simulink model "Energisense"  (R2025a)
settings: Solver=VariableStepAuto  StartTime=0.0  StopTime=100  RelTol=1e-3
settings Model: Creator=Aryan  LastModifiedBy=Aryan

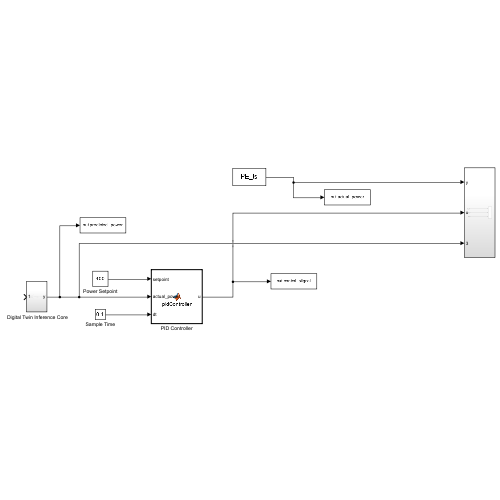
[thumbnail: Simulink's stored preview of the top-level diagram]
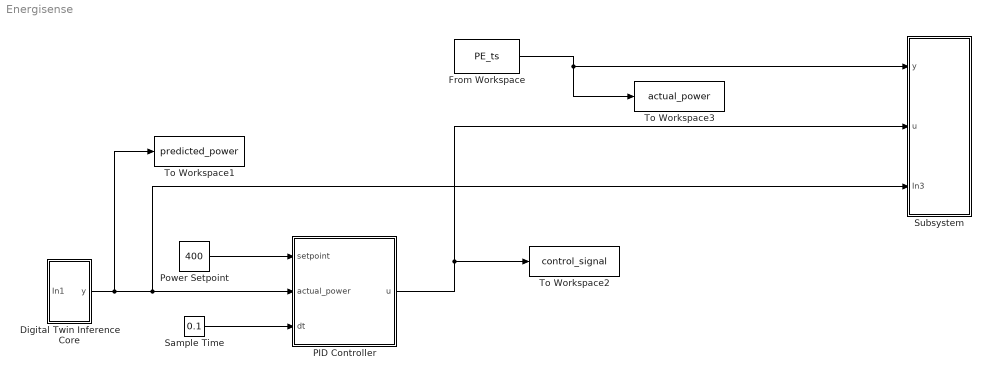
== system Energisense ==
  " Digital Twin Inference Core " : Subsystem
  From Workspace : FromWorkspace  VariableName=PE_ts  OutDataTypeStr=double
  PID Controller : MATLAB Function  TreatAsAtomicUnit=on
  Power Setpoint : Constant  Value=400
  Sample Time : Constant  Value=0.1
  Subsystem : Subsystem
  To Workspace1 : ToWorkspace  VariableName=predicted_power  SampleTime=-1
  To Workspace2 : ToWorkspace  VariableName=control_signal  SampleTime=-1
  To Workspace3 : ToWorkspace  VariableName=actual_power  SampleTime=-1
  wires:
  Sample Time/1 -> PID Controller/3(dt)
  Power Setpoint/1 -> PID Controller/1(setpoint)
  " Digital Twin Inference Core "/1(y) -> To Workspace1/1, Subsystem/3(In3), PID Controller/2(actual_power)
  PID Controller/1(u) -> Subsystem/2(u), To Workspace2/1
  From Workspace/1 -> Subsystem/1(y), To Workspace3/1

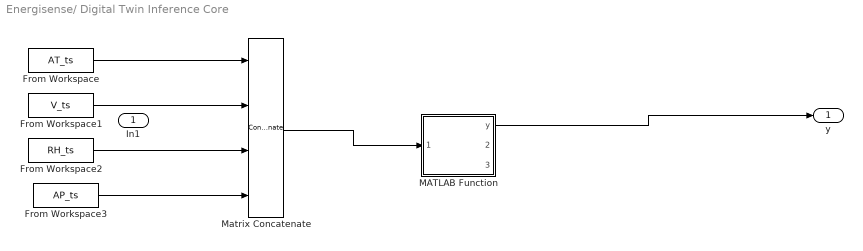
== system Energisense/ Digital Twin Inference Core  ==
  In1 : Inport
  From Workspace : FromWorkspace  VariableName=AT_ts  OutDataTypeStr=double
  From Workspace1 : FromWorkspace  VariableName=V_ts  OutDataTypeStr=double
  From Workspace2 : FromWorkspace  VariableName=RH_ts  OutDataTypeStr=double
  From Workspace3 : FromWorkspace  VariableName=AP_ts  OutDataTypeStr=double
  MATLAB Function : MATLAB Function  TreatAsAtomicUnit=on
  Matrix Concatenate : Concatenate  NumInputs=4  ConcatenateDimension=2
  y : Outport
  wires:
  Matrix Concatenate/1 -> MATLAB Function/1(input_vector)
  From Workspace2/1 -> Matrix Concatenate/3
  From Workspace1/1 -> Matrix Concatenate/2
  From Workspace/1 -> Matrix Concatenate/1
  MATLAB Function/1(y) -> y/1
  From Workspace3/1 -> Matrix Concatenate/4

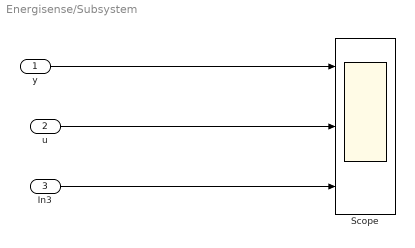
== system Energisense/Subsystem ==
  y : Inport
  u : Inport  Port=2
  In3 : Inport  Port=3
  Scope : Scope  NumInputPorts=3
      settings: Title=Predicted Vs Actual PE  ActiveDisplayYMinimum=-941.66758948423035  ActiveDisplayYMaximum=2122.0302698165196  YLabel=PE  DataLoggingVariableName=Predicted_VS_Actual
  wires:
  y/1 -> Scope/1
  u/1 -> Scope/2
  In3/1 -> Scope/3

== matlab function Energisense/PID Controller ==
  data: setpoint input; u output; actual_power input; dt input
function u = pidController(setpoint, actual_power, dt)
%#codegen
% PID Controller for Power Regulation
% 
% Inputs:
%   setpoint - Desired power output (scalar double)
%   actual_power - Current actual power (scalar double) 
%   dt - Sample time in seconds (scalar double)
%
% Outputs:
%   u - Control signal (scalar double)

    % Declare persistent variables for integral and derivative terms
    persistent integral_error previous_error initialized;
    
    % Initialize persistent variables
    if isempty(initialized)
        integral_error = 0.0;
        previous_error = 0.0;
        initialized = true;
    end
    
    % PID Controller Parameters (Tunable - adjust these for your system)
    Kp = 1.5;      % Proportional gain
    Ki = 0.1;      % Integral gain  
    Kd = 0.05;     % Derivative gain
    
    % Control signal limits
    u_max = 100.0;  % Maximum control signal
    u_min = -100.0; % Minimum control signal
    
    % Calculate error
    error = setpoint - actual_power;
    
    % Proportional term
    P_term = Kp * error;
    
    % Integral term (with sample time)
    integral_error = integral_error + error * dt;
    I_term = Ki * integral_error;
    
    % Derivative term (with sample time) 
    if dt > 0
        derivative_error = (error - previous_error) / dt;
    else
        derivative_error = 0;
    end
    D_term = Kd * derivative_error;
    
    % Calculate PID output
    u = P_term + I_term + D_term;
    
    % Apply control signal limits (saturation)
    u_saturated = u;
    if u > u_max
        u_saturated = u_max;
    elseif u < u_min
        u_saturated = u_min;
    end
    
    % Anti-windup: Reset integral if control signal is saturated
    if (u ~= u_saturated) && (sign(error) == sign(integral_error))
        integral_error = integral_error - error * dt;
    end
    
    % Store error for next iteration
    previous_error = error;
    
    % Output saturated control signal
    u = u_saturated;
    
    % Ensure output is scalar double
    u = double(u);
end

== matlab function Energisense/ Digital Twin Inference Core /MATLAB Function ==
  data: input_vector input; y output; confidence output; anomaly_flag output
function [y, confidence, anomaly_flag] = fcn(input_vector)
%#codegen
% Digital Twin - Complete CCPP Model with Bias Correction

    % Extract scalars from input vector
    if numel(input_vector) >= 4
        AT = double(input_vector(1));  % Ambient Temperature
        V = double(input_vector(2));   % Vacuum
        RH = double(input_vector(3));  % Relative Humidity  
        AP = double(input_vector(4));  % Atmospheric Pressure
    else
        % Default values if input is wrong size
        AT = 20.0;
        V = 40.0;
        RH = 70.0;
        AP = 1013.0;
    end
    
    % Input validation
    input_valid = true;
    if isnan(AT) || isnan(V) || isnan(RH) || isnan(AP) || ...
       isinf(AT) || isinf(V) || isinf(RH) || isinf(AP) || ...
       (AT < -50.0) || (AT > 100.0) || (V < 0.0) || (V > 200.0) || ...
       (RH < 0.0) || (RH > 150.0) || (AP < 900.0) || (AP > 1100.0)
        input_valid = false;
    end
    
    if input_valid
        % COMPLETE CCPP PHYSICS MODEL
        base_power = 454.5;
        
        % Primary linear effects (most important)
        temp_effect = -2.2 * AT;       % Temperature impact
        vacuum_effect = -0.39 * V;     % Vacuum impact  
        humidity_effect = -0.078 * RH; % Humidity impact
        pressure_effect = 0.043 * AP;  % Pressure impact
        
        % Interaction effects (ensemble model characteristics)
        AT_V_int = 0.0086 * AT * V;
        AT_RH_int = 0.0021 * AT * RH;
        V_RH_int = 0.0012 * V * RH;
        AT_AP_int = 0.0018 * AT * AP;
        
        % Non-linear effects (polynomial terms)
        AT_sq = -0.0189 * AT * AT;
        V_sq = -0.0067 * V * V;
        RH_sq = -0.0003 * RH * RH;
        
        % Higher-order interactions (ensemble specialty)
        three_way_1 = 0.000043 * AT * V * RH;
        three_way_2 = 0.000028 * AT * V * AP;
        
        % Threshold effects (decision tree characteristics)
        threshold_adj = 0.0;
        if AT > 20.0
            threshold_adj = threshold_adj - 0.5 * (AT - 20.0);
        end
        if V > 50.0
            threshold_adj = threshold_adj - 0.3 * (V - 50.0);
        end
        
        % FIXED BIAS CORRECTION (was 2.0, now 27.0)
        bias_correction = 27.0;  % Corrects the 26.4 MW systematic error
        
        % Calculate total power output
        y = base_power + temp_effect + vacuum_effect + humidity_effect + pressure_effect + ...
            AT_V_int + AT_RH_int + V_RH_int + AT_AP_int + ...
            AT_sq + V_sq + RH_sq + three_way_1 + three_way_2 + ...
            threshold_adj + bias_correction;
        
        % DYNAMIC CONFIDENCE CALCULATION
        % Higher confidence when closer to optimal conditions
        AT_optimal = 15.0;
        V_optimal = 40.0; 
        RH_optimal = 60.0;
        AP_optimal = 1013.0;
        
        % Operating ranges for confidence calculation
        AT_range = 35.3;  % Full operating range
        V_range = 56.2;
        RH_range = 74.6;
        AP_range = 40.41;
        
        % Distance-based confidence (closer to optimal = higher confidence)
        AT_conf = 1.0 - 0.8 * abs(AT - AT_optimal) / AT_range;
        V_conf = 1.0 - 0.6 * abs(V - V_optimal) / V_range;
        RH_conf = 1.0 - 0.3 * abs(RH - RH_optimal) / RH_range;
        AP_conf = 1.0 - 0.2 * abs(AP - AP_optimal) / AP_range;
        
        % Weighted confidence (AT and V most important in CCPP)
        confidence = 0.4 * AT_conf + 0.3 * V_conf + 0.2 * RH_conf + 0.1 * AP_conf;
        
        % ANOMALY DETECTION - check operating envelope
        AT_ok = (AT >= 1.81) && (AT <= 37.11);
        V_ok = (V >= 25.36) && (V <= 81.56);
        RH_ok = (RH >= 25.56) && (RH <= 100.16);
        AP_ok = (AP >= 992.89) && (AP <= 1033.30);
        
        anomaly_flag = ~(AT_ok && V_ok && RH_ok && AP_ok);
        
        % Reduce confidence if anomaly detected
        if anomaly_flag
            confidence = confidence * 0.5;
        end
        
    else
        % Invalid inputs - safe defaults
        y = 450.0;
        confidence = 0.1;
        anomaly_flag = true;
    end
    
    % Final bounds and type conversion
    y = max(400.0, min(500.0, y));
    confidence = max(0.1, min(1.0, confidence));
    
    % Ensure scalar outputs for Simulink
    y = double(y);
    confidence = double(confidence);
    anomaly_flag = logical(anomaly_flag);
end
